simulink model "RobotControl"  (R2016b)
settings: Solver=FixedStepDiscrete  StartTime=0.0  StopTime=inf  FixedStep=0.001  RelTol=1e-3
libraries: arduinolib x9, RobotControlLib x1
settings Model: ExtModeTrigDuration=2  Creator=oelkawok  LastModifiedBy=oelkawok
settings DataIOCC: SaveOutput=off  SaveTime=off
settings OptimizationCC: DefaultParameterBehavior=Inlined  UseFloatMulNetSlope=on  DefaultUnderspecifiedDataType=single  EfficientFloat2IntCast=on  MaxStackSize=64
settings HardwareCC: ProdBitPerInt=16  ProdBitPerPointer=16  ProdBitPerSizeT=16  ProdBitPerPtrDiffT=16  ProdLargestAtomicFloat=None  ProdWordSize=8  ProdHWDeviceType=Atmel->AVR  UseEmbeddedCoderFeatures=off
settings SFSimCC: SimUserSources="\"twi.c\""
settings RTWCC: SystemTargetFile=ert.tlc  GenerateMakefile=off  TemplateMakefile=RTW.MSVCBuild  Description=Create Visual C/C++ Solution File for Embedded Coder  GenerateReport=on  RTWUseSimCustomCode=on  CustomSource="\"twi.c\""  Toolchain=Arduino AVR  BuildConfiguration=Faster Runs  IncludeHyperlinkInReport=on  LaunchReport=on  GenerateTraceInfo=on  GenerateTraceReport=on  GenerateTraceReportSl=on  GenerateTraceReportSf=on  GenerateTraceReportEml=on  GenerateCodeMetricsReport=on
settings CodeAppCC: ForceParamTrailComments=on  IgnoreCustomStorageClasses=off  OperatorAnnotations=on  SimulinkDataObjDesc=on  SFDataObjDesc=on  MATLABFcnDesc=on  InsertBlockDesc=on  MATLABSourceComments=on
settings ERTTargetCC: GenerateSampleERTMain=on  SupportComplex=off  InlinedParameterPlacement=NonHierarchical  ERTCustomFileTemplate=example_file_process.tlc  MemSecPackage=Simulink

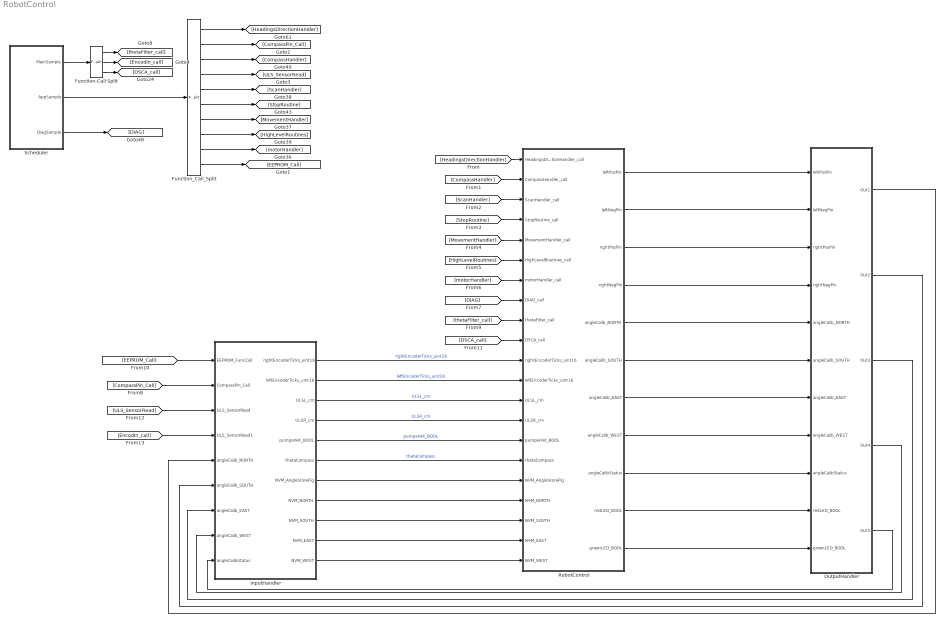
== system RobotControl ==
  Function-Call Split : FunctionCallSplit  IconShape=distinctive  NumOutputPorts=3  OutputPortLayout=default
  Function_Call_Split : FunctionCallSplit  IconShape=distinctive  NumOutputPorts=10  OutputPortLayout=default
  InputHandler : Subsystem
  OutputHandler : Subsystem
  RobotControl : Subsystem
  Scheduler : Subsystem
  wires:
  Scheduler/2(AppSample) -> Function_Call_Split/1
  Function_Call_Split/1 -> [HeadingsDirectionHandler]
  Scheduler/3(DiagSample) -> [DIAG]
  [HeadingsDirectionHandler] -> RobotControl/1(HeadingsDirectionHandler_call)
  [CompassHandler] -> RobotControl/2(CompassHandler_call)
  [ScanHandler] -> RobotControl/3(ScanHandler_call)
  [StopRoutine] -> RobotControl/4(StopRoutine_call)
  [HighLevelRoutines] -> RobotControl/6(HighLevelRoutines_call)
  [MovementHandler] -> RobotControl/5(MovementHandler_call)
  [motorHandler] -> RobotControl/7(motorHandler_call)
  RobotControl/1(leftPosPin) -> OutputHandler/1(leftPosPin)
  RobotControl/2(leftNegPin) -> OutputHandler/2(leftNegPin)
  RobotControl/3(rightPosPin) -> OutputHandler/3(rightPosPin)
  RobotControl/4(rightNegPin) -> OutputHandler/4(rightNegPin)
  RobotControl/5(angleCalib_NORTH) -> OutputHandler/5(angleCalib_NORTH)
  RobotControl/6(angleCalib_SOUTH) -> OutputHandler/6(angleCalib_SOUTH)
  RobotControl/7(angleCalib_EAST) -> OutputHandler/7(angleCalib_EAST)
  RobotControl/8(angleCalib_WEST) -> OutputHandler/8(angleCalib_WEST)
  RobotControl/9(angleCalibStatus) -> OutputHandler/9(angleCalibStatus)
  RobotControl/10(redLED_BOOL) -> OutputHandler/10(redLED_BOOL)
  RobotControl/11(greenLED_BOOL) -> OutputHandler/11(greenLED_BOOL)
  [DIAG] -> RobotControl/8(DIAG_call)
  [EEPROM_Call] -> InputHandler/1(EEPROM_FuncCall)
  OutputHandler/5(Out5) -> InputHandler/9(angleCalibStatus)
  OutputHandler/4(Out4) -> InputHandler/8(angleCalib_WEST)
  OutputHandler/3(Out3) -> InputHandler/7(angleCalib_EAST)
  OutputHandler/2(Out2) -> InputHandler/6(angleCalib_SOUTH)
  OutputHandler/1(Out1) -> InputHandler/5(angleCalib_NORTH)
  [CompassPin_Call] -> InputHandler/2(CompassPin_Call)
  Function_Call_Split/2 -> [CompassPin_Call]
  Function_Call_Split/3 -> [CompassHandler]
  Scheduler/1(MainSample) -> Function-Call Split/1
  Function-Call Split/1 -> [thetaFilter_call]
  [DSCA_call] -> RobotControl/10(DSCA_call)
  [thetaFilter_call] -> RobotControl/9(thetaFilter_call)
  InputHandler/11(NVM_WEST) -> RobotControl/21(NVM_WEST)
  InputHandler/10(NVM_EAST) -> RobotControl/20(NVM_EAST)
  InputHandler/9(NVM_SOUTH) -> RobotControl/19(NVM_SOUTH)
  InputHandler/8(NVM_NORTH) -> RobotControl/18(NVM_NORTH)
  InputHandler/7(NVM_AngleStoreFlg) -> RobotControl/17(NVM_AngleStoreFlg)
  InputHandler/6(thetaCompass) -> RobotControl/16(thetaCompass)  "thetaCompass"
  InputHandler/5(pumperHit_BOOL) -> RobotControl/15(pumperHit_BOOL)  "pumperHit_BOOL"
  InputHandler/4(ULSR_cm) -> RobotControl/14(ULSR_cm)  "ULSR_cm"
  InputHandler/3(ULSL_cm) -> RobotControl/13(ULSL_cm)  "ULSL_cm"
  InputHandler/2(leftEncoderTicks_uint16) -> RobotControl/12(leftEncoderTicks_uint16)  "leftEncoderTicks_uint16"
  InputHandler/1(rightEncoderTicks_uint16) -> RobotControl/11(rightEncoderTicks_uint16)  "rightEncoderTicks_uint16"
  Function_Call_Split/4 -> [ULS_SensorRead]
  Function_Call_Split/5 -> [ScanHandler]
  Function_Call_Split/7 -> [MovementHandler]
  Function_Call_Split/6 -> [StopRoutine]
  Function_Call_Split/8 -> [HighLevelRoutines]
  Function_Call_Split/9 -> [motorHandler]
  Function_Call_Split/10 -> [EEPROM_Call]
  [ULS_SensorRead] -> InputHandler/3(ULS_SensorRead)
  Function-Call Split/3 -> [DSCA_call]
  Function-Call Split/2 -> [EncodIn_call]
  [EncodIn_call] -> InputHandler/4(ULS_SensorRead1)

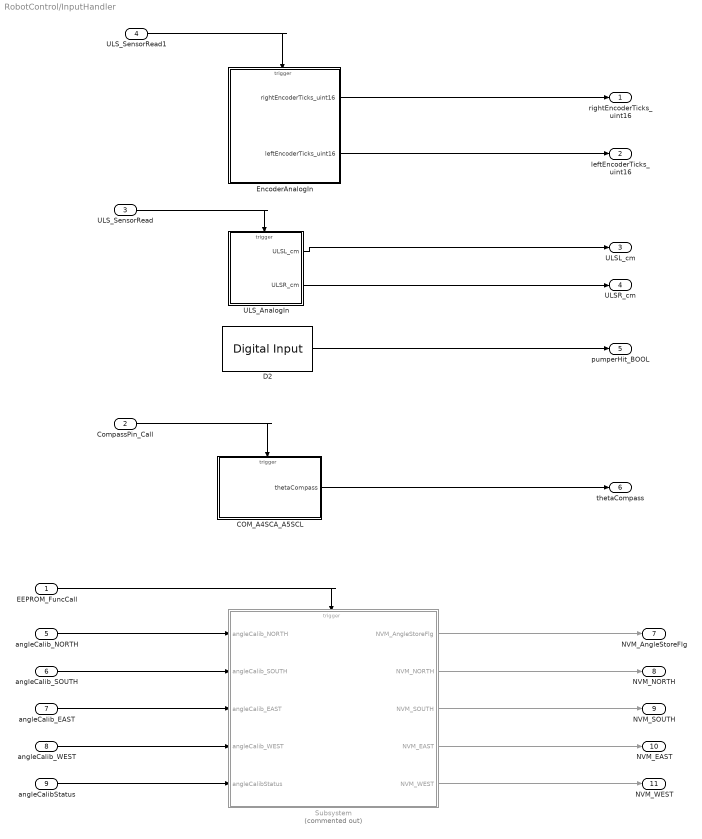
== system RobotControl/InputHandler ==
  EEPROM_FuncCall : Inport
  CompassPin_Call : Inport  Port=2
  ULS_SensorRead : Inport  Port=3
  ULS_SensorRead1 : Inport  Port=4
  angleCalib_NORTH : Inport  Port=5
  angleCalib_SOUTH : Inport  Port=6
  angleCalib_EAST : Inport  Port=7
  angleCalib_WEST : Inport  Port=8
  angleCalibStatus : Inport  Port=9
  COM_A4SCA_A5SCL : Subsystem
      settings: RTWSystemCode=Nonreusable function  RTWFcnNameOpts=Use subsystem name  RTWFileNameOpts=Use subsystem name
  D2 : arduinolib/Digital Input  pinNumber=2  sampleTime=-1  blockPlatform=arduino
  EncoderAnalogIn : Subsystem  RTWFileName=DSCA
      settings: RTWSystemCode=Nonreusable function  RTWFcnNameOpts=Use subsystem name  RTWFileNameOpts=User specified
  Subsystem : Subsystem  Commented=on
  ULS_AnalogIn : Subsystem  RTWFileName=ScanHandler
      settings: ErrorFcn=ScanHandler  RTWSystemCode=Nonreusable function  RTWFcnNameOpts=Use subsystem name  RTWFileNameOpts=User specified
  rightEncoderTicks_uint16 : Outport
  leftEncoderTicks_uint16 : Outport  Port=2
  ULSL_cm : Outport  Port=3
  ULSR_cm : Outport  Port=4
  pumperHit_BOOL : Outport  Port=5
  thetaCompass : Outport  Port=6
  NVM_AngleStoreFlg : Outport  Port=7
  NVM_NORTH : Outport  Port=8
  NVM_SOUTH : Outport  Port=9
  NVM_EAST : Outport  Port=10
  NVM_WEST : Outport  Port=11
  wires:
  D2/1 -> pumperHit_BOOL/1
  EEPROM_FuncCall/1 -> Subsystem/Trigger
  angleCalib_NORTH/1 -> Subsystem/1(angleCalib_NORTH)
  angleCalib_SOUTH/1 -> Subsystem/2(angleCalib_SOUTH)
  angleCalib_EAST/1 -> Subsystem/3(angleCalib_EAST)
  angleCalibStatus/1 -> Subsystem/5(angleCalibStatus)
  angleCalib_WEST/1 -> Subsystem/4(angleCalib_WEST)
  Subsystem/5(NVM_WEST) -> NVM_WEST/1
  Subsystem/4(NVM_EAST) -> NVM_EAST/1
  Subsystem/3(NVM_SOUTH) -> NVM_SOUTH/1
  Subsystem/1(NVM_AngleStoreFlg) -> NVM_AngleStoreFlg/1
  Subsystem/2(NVM_NORTH) -> NVM_NORTH/1
  COM_A4SCA_A5SCL/1(thetaCompass) -> thetaCompass/1
  CompassPin_Call/1 -> COM_A4SCA_A5SCL/Trigger
  ULS_AnalogIn/1(ULSL_cm) -> ULSL_cm/1
  ULS_AnalogIn/2(ULSR_cm) -> ULSR_cm/1
  ULS_SensorRead/1 -> ULS_AnalogIn/Trigger
  EncoderAnalogIn/1(rightEncoderTicks_uint16) -> rightEncoderTicks_uint16/1
  EncoderAnalogIn/2(leftEncoderTicks_uint16) -> leftEncoderTicks_uint16/1
  ULS_SensorRead1/1 -> EncoderAnalogIn/Trigger

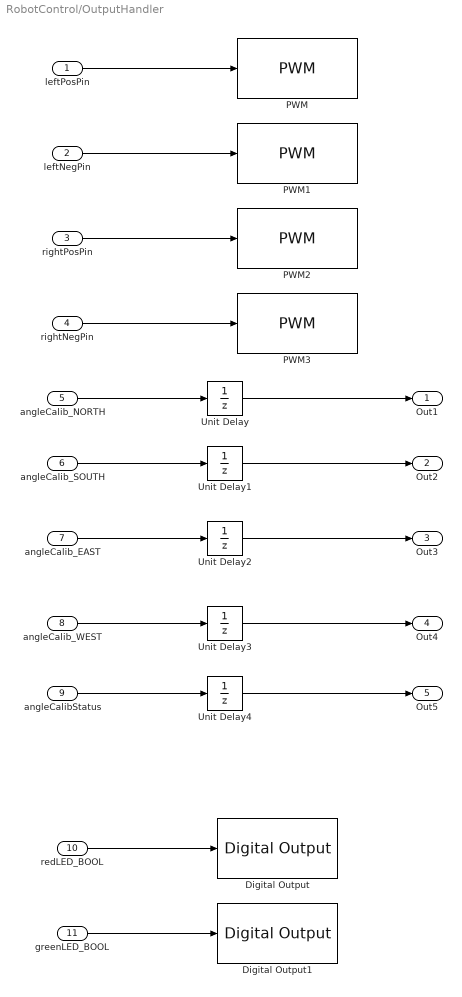
== system RobotControl/OutputHandler ==
  leftPosPin : Inport
  leftNegPin : Inport  Port=2
  rightPosPin : Inport  Port=3
  rightNegPin : Inport  Port=4
  angleCalib_NORTH : Inport  Port=5
  angleCalib_SOUTH : Inport  Port=6
  angleCalib_EAST : Inport  Port=7
  angleCalib_WEST : Inport  Port=8
  angleCalibStatus : Inport  Port=9
  redLED_BOOL : Inport  Port=10
  greenLED_BOOL : Inport  Port=11
  Digital Output : arduinolib/Digital Output  pinNumber=3  blockPlatform=arduino
  Digital Output1 : arduinolib/Digital Output  pinNumber=11  blockPlatform=arduino
  PWM : arduinolib/PWM  pinNumber=5  blockPlatform=arduino
  PWM1 : arduinolib/PWM  pinNumber=6  blockPlatform=arduino
  PWM2 : arduinolib/PWM  pinNumber=9  blockPlatform=arduino
  PWM3 : arduinolib/PWM  pinNumber=10  blockPlatform=arduino
  Unit Delay{,1..4} (5 alike) : UnitDelay  SampleTime=-1
  Out1 : Outport
  Out2 : Outport  Port=2
  Out3 : Outport  Port=3
  Out4 : Outport  Port=4
  Out5 : Outport  Port=5
  wires:
  angleCalib_NORTH/1 -> Unit Delay/1
  angleCalib_SOUTH/1 -> Unit Delay1/1
  angleCalib_WEST/1 -> Unit Delay3/1
  angleCalib_EAST/1 -> Unit Delay2/1
  angleCalibStatus/1 -> Unit Delay4/1
  Unit Delay/1 -> Out1/1
  Unit Delay1/1 -> Out2/1
  Unit Delay3/1 -> Out4/1
  Unit Delay2/1 -> Out3/1
  Unit Delay4/1 -> Out5/1
  leftPosPin/1 -> PWM/1
  leftNegPin/1 -> PWM1/1
  rightPosPin/1 -> PWM2/1
  rightNegPin/1 -> PWM3/1
  redLED_BOOL/1 -> Digital Output/1
  greenLED_BOOL/1 -> Digital Output1/1

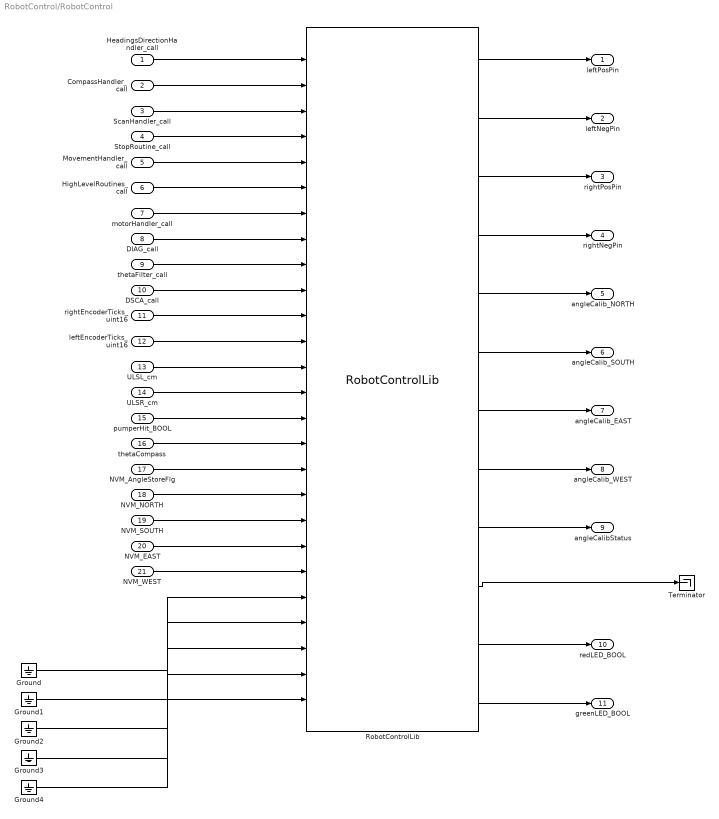
== system RobotControl/RobotControl ==
  HeadingsDirectionHandler_call : Inport  PortDimensions=1
  CompassHandler_call : Inport  Port=2  PortDimensions=1
  ScanHandler_call : Inport  Port=3  PortDimensions=1
  StopRoutine_call : Inport  Port=4  PortDimensions=1
  MovementHandler_call : Inport  Port=5  PortDimensions=1
  HighLevelRoutines_call : Inport  Port=6  PortDimensions=1
  motorHandler_call : Inport  Port=7  PortDimensions=1
  DIAG_call : Inport  Port=8  PortDimensions=1
  thetaFilter_call : Inport  Port=9  PortDimensions=1
  DSCA_call : Inport  Port=10  PortDimensions=1
  rightEncoderTicks_uint16 : Inport  Port=11  PortDimensions=1
  leftEncoderTicks_uint16 : Inport  Port=12  PortDimensions=1
  ULSL_cm : Inport  Port=13  PortDimensions=1
  ULSR_cm : Inport  Port=14  PortDimensions=1
  pumperHit_BOOL : Inport  Port=15  OutDataTypeStr=boolean  PortDimensions=1
  thetaCompass : Inport  Port=16  OutDataTypeStr=int16  PortDimensions=1
  NVM_AngleStoreFlg : Inport  Port=17  PortDimensions=1
  NVM_NORTH : Inport  Port=18  PortDimensions=1
  NVM_SOUTH : Inport  Port=19  PortDimensions=1
  NVM_EAST : Inport  Port=20  PortDimensions=1
  NVM_WEST : Inport  Port=21  PortDimensions=1
  Ground{,1..4} (5 alike) : Ground
  RobotControlLib : RobotControlLib/RobotControlLib
  Terminator : Terminator
  leftPosPin : Outport  OutDataTypeStr=uint8  PortDimensions=1
      settings: AttributesFormatString=|
      | Mode: %<OutputWhenDisabled>
      | Init: %<InitialOutput>
  leftNegPin : Outport  Port=2  OutDataTypeStr=uint8  PortDimensions=1
      settings: AttributesFormatString=|
      | Mode: %<OutputWhenDisabled>
      | Init: %<InitialOutput>
  rightPosPin : Outport  Port=3  OutDataTypeStr=uint8  PortDimensions=1
      settings: AttributesFormatString=|
      | Mode: %<OutputWhenDisabled>
      | Init: %<InitialOutput>
  rightNegPin : Outport  Port=4  OutDataTypeStr=uint8  PortDimensions=1
      settings: AttributesFormatString=|
      | Mode: %<OutputWhenDisabled>
      | Init: %<InitialOutput>
  angleCalib_NORTH : Outport  Port=5  InitialOutput=0
      settings: AttributesFormatString=|
      | Mode: %<OutputWhenDisabled>
      | Init: %<InitialOutput>
  angleCalib_SOUTH : Outport  Port=6  InitialOutput=0
      settings: AttributesFormatString=|
      | Mode: %<OutputWhenDisabled>
      | Init: %<InitialOutput>
  angleCalib_EAST : Outport  Port=7  InitialOutput=0
      settings: AttributesFormatString=|
      | Mode: %<OutputWhenDisabled>
      | Init: %<InitialOutput>
  angleCalib_WEST : Outport  Port=8  InitialOutput=0
      settings: AttributesFormatString=|
      | Mode: %<OutputWhenDisabled>
      | Init: %<InitialOutput>
  angleCalibStatus : Outport  Port=9
      settings: AttributesFormatString=|
      | Mode: %<OutputWhenDisabled>
      | Init: %<InitialOutput>
  redLED_BOOL : Outport  Port=10
      settings: AttributesFormatString=|
      | Mode: %<OutputWhenDisabled>
      | Init: %<InitialOutput>
  greenLED_BOOL : Outport  Port=11
      settings: AttributesFormatString=|
      | Mode: %<OutputWhenDisabled>
      | Init: %<InitialOutput>
  wires:
  RobotControlLib/5 -> angleCalib_NORTH/1
  RobotControlLib/6 -> angleCalib_SOUTH/1
  RobotControlLib/7 -> angleCalib_EAST/1
  RobotControlLib/8 -> angleCalib_WEST/1
  RobotControlLib/4 -> rightNegPin/1
  RobotControlLib/3 -> rightPosPin/1
  RobotControlLib/2 -> leftNegPin/1
  RobotControlLib/1 -> leftPosPin/1
  RobotControlLib/11 -> redLED_BOOL/1
  RobotControlLib/12 -> greenLED_BOOL/1
  RobotControlLib/9 -> angleCalibStatus/1
  RobotControlLib/10 -> Terminator/1
  ScanHandler_call/1 -> RobotControlLib/3
  CompassHandler_call/1 -> RobotControlLib/2
  StopRoutine_call/1 -> RobotControlLib/4
  HeadingsDirectionHandler_call/1 -> RobotControlLib/1
  MovementHandler_call/1 -> RobotControlLib/5
  HighLevelRoutines_call/1 -> RobotControlLib/6
  motorHandler_call/1 -> RobotControlLib/7
  DIAG_call/1 -> RobotControlLib/8
  thetaFilter_call/1 -> RobotControlLib/9
  DSCA_call/1 -> RobotControlLib/10
  rightEncoderTicks_uint16/1 -> RobotControlLib/11
  leftEncoderTicks_uint16/1 -> RobotControlLib/12
  ULSL_cm/1 -> RobotControlLib/13
  ULSR_cm/1 -> RobotControlLib/14
  pumperHit_BOOL/1 -> RobotControlLib/15
  thetaCompass/1 -> RobotControlLib/16
  NVM_AngleStoreFlg/1 -> RobotControlLib/17
  NVM_NORTH/1 -> RobotControlLib/18
  NVM_SOUTH/1 -> RobotControlLib/19
  NVM_EAST/1 -> RobotControlLib/20
  NVM_WEST/1 -> RobotControlLib/21
  Ground/1 -> RobotControlLib/22
  Ground1/1 -> RobotControlLib/23
  Ground2/1 -> RobotControlLib/24
  Ground3/1 -> RobotControlLib/25
  Ground4/1 -> RobotControlLib/26

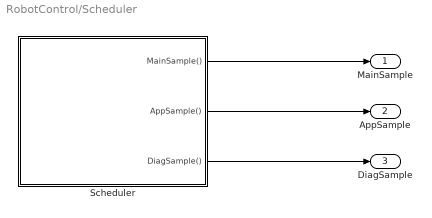
== system RobotControl/Scheduler ==
  Scheduler : Stateflow chart  TreatAsAtomicUnit=on
  MainSample : Outport
  AppSample : Outport  Port=2
  DiagSample : Outport  Port=3
  wires:
  Scheduler/3(DiagSample()) -> DiagSample/1
  Scheduler/2(AppSample()) -> AppSample/1
  Scheduler/1(MainSample()) -> MainSample/1

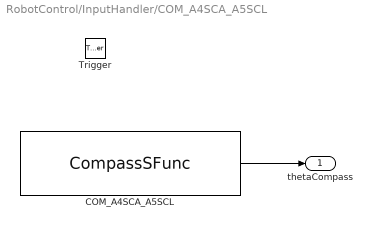
== system RobotControl/InputHandler/COM_A4SCA_A5SCL ==
  Trigger : TriggerPort  TriggerType=function-call  VariantControl=Variant  PortDimensions=1
  COM_A4SCA_A5SCL : S-Function  InitFcn=try, set_param(gcb,'FunctionName','CompassSFunc'), end  FunctionName=CompassSFunc  SFunctionModules=CompassSFunc_wrapper  SFunctionDeploymentMode=off  EnableBusSupport=off  mask(S-Function Builder){}
      mask help: Simulink:masks:SFunctionBuilder_MD
      mask init:
      | val = [[.9  0.75 0.75 1 1 .9 .9 1]',[1 1 0.75 0.75 .9 .9 1 .9]'];try , sys = get_param(gcb,'SfunBuilderFcnName');if isempty(sys), sys = get_param(gcb,'FunctionName'); end,catch, sys = get_param(gcb,'FunctionName'); end
      settings: CopyFcn=set_param(gcbh,'LinkStatus','none')  PreSaveFcn=try, set_param(gcb,'FunctionName','CompassSFunc'), end  OpenFcn=sfunctionwizard(gcbh)
      mask Display: plot(val(:,1),val(:,2)),disp(sys), port_label('output',1,'Temp_angle')
  thetaCompass : Outport
  wires:
  COM_A4SCA_A5SCL/1 -> thetaCompass/1

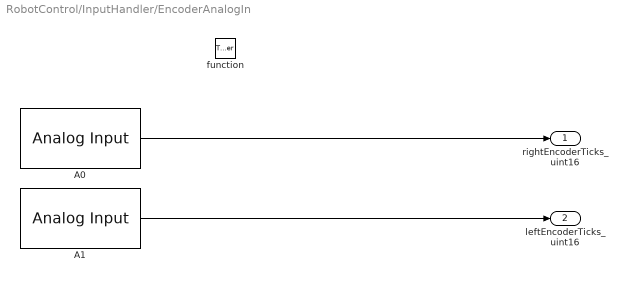
== system RobotControl/InputHandler/EncoderAnalogIn ==
  function : TriggerPort  TriggerType=function-call  VariantControl=Variant
  A0 : arduinolib/Analog Input  pinNumber=0  sampleTime=-1  blockPlatform=arduino
  A1 : arduinolib/Analog Input  pinNumber=1  sampleTime=-1  blockPlatform=arduino
  rightEncoderTicks_uint16 : Outport
  leftEncoderTicks_uint16 : Outport  Port=2
  wires:
  A1/1 -> leftEncoderTicks_uint16/1
  A0/1 -> rightEncoderTicks_uint16/1

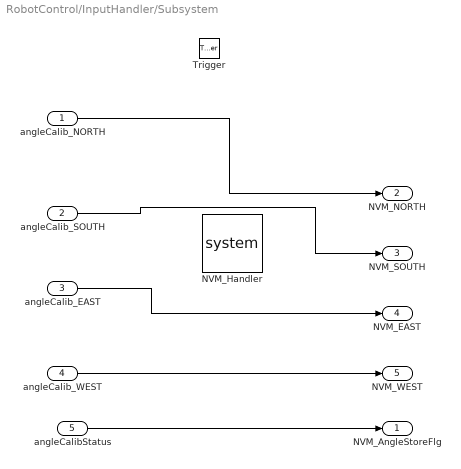
== system RobotControl/InputHandler/Subsystem ==
  angleCalib_NORTH : Inport
  angleCalib_SOUTH : Inport  Port=2
  angleCalib_EAST : Inport  Port=3
  angleCalib_WEST : Inport  Port=4
  angleCalibStatus : Inport  Port=5
  Trigger : TriggerPort  TriggerType=function-call  VariantControl=Variant  PortDimensions=1
  NVM_Handler : S-Function  SFunctionDeploymentMode=off  EnableBusSupport=off  mask(S-Function Builder){}
      mask help: Simulink:masks:SFunctionBuilder_MD
      mask init:
      | val = [[.9  0.75 0.75 1 1 .9 .9 1]',[1 1 0.75 0.75 .9 .9 1 .9]'];
      | sys = get_param(gcbh,'FunctionName');
      settings: CopyFcn=set_param(gcbh,'LinkStatus','none')  OpenFcn=sfunctionwizard(gcbh)
      mask Display:
      | plot(val(:,1),val(:,2))
      | disp(sys)
  NVM_AngleStoreFlg : Outport
  NVM_NORTH : Outport  Port=2
  NVM_SOUTH : Outport  Port=3
  NVM_EAST : Outport  Port=4
  NVM_WEST : Outport  Port=5
  wires:
  angleCalib_NORTH/1 -> NVM_NORTH/1
  angleCalib_SOUTH/1 -> NVM_SOUTH/1
  angleCalib_EAST/1 -> NVM_EAST/1
  angleCalib_WEST/1 -> NVM_WEST/1
  angleCalibStatus/1 -> NVM_AngleStoreFlg/1

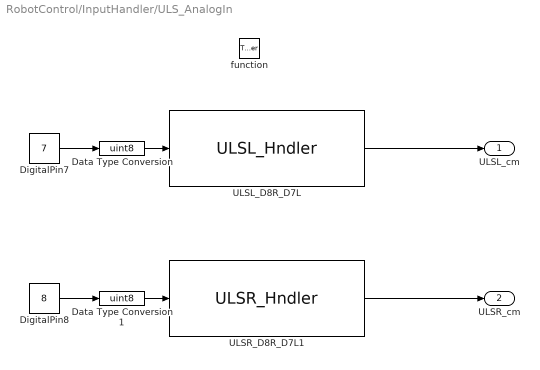
== system RobotControl/InputHandler/ULS_AnalogIn ==
  function : TriggerPort  TriggerType=function-call  VariantControl=Variant
  Data Type Conversion : DataTypeConversion  OutDataTypeStr=uint8
  Data Type Conversion1 : DataTypeConversion  OutDataTypeStr=uint8
  DigitalPin7 : Constant  Value=7
  DigitalPin8 : Constant  Value=8
  ULSL_D8R_D7L : S-Function  InitFcn=try, set_param(gcb,'FunctionName','ULSL_Hndler'), end  FunctionName=ULSL_Hndler  SFunctionModules=ULSL_Hndler_wrapper  SFunctionDeploymentMode=off  EnableBusSupport=off  mask(S-Function Builder){}
      mask help: Simulink:masks:SFunctionBuilder_MD
      mask init: same as RobotControl/InputHandler/COM_A4SCA_A5SCL/COM_A4SCA_A5SCL
      settings: CopyFcn=set_param(gcbh,'LinkStatus','none')  PreSaveFcn=try, set_param(gcb,'FunctionName','ULSL_Hndler'), end  OpenFcn=sfunctionwizard(gcbh)
      mask Display: plot(val(:,1),val(:,2)),disp(sys), port_label('input',1,'ULSL_Pin'), port_label('output',1,'ULSL_cm')
  ULSR_D8R_D7L1 : S-Function  InitFcn=try, set_param(gcb,'FunctionName','ULSR_Hndler'), end  FunctionName=ULSR_Hndler  SFunctionModules=ULSR_Hndler_wrapper  SFunctionDeploymentMode=off  EnableBusSupport=off  mask(S-Function Builder){}
      mask help: Simulink:masks:SFunctionBuilder_MD
      mask init: same as RobotControl/InputHandler/COM_A4SCA_A5SCL/COM_A4SCA_A5SCL
      settings: CopyFcn=set_param(gcbh,'LinkStatus','none')  PreSaveFcn=try, set_param(gcb,'FunctionName','ULSR_Hndler'), end  OpenFcn=sfunctionwizard(gcbh)
      mask Display: plot(val(:,1),val(:,2)),disp(sys), port_label('input',1,'ULSR_Pin'), port_label('output',1,'ULSR_cm')
  ULSL_cm : Outport
  ULSR_cm : Outport  Port=2
  wires:
  ULSL_D8R_D7L/1 -> ULSL_cm/1
  Data Type Conversion1/1 -> ULSR_D8R_D7L1/1
  DigitalPin7/1 -> Data Type Conversion/1
  DigitalPin8/1 -> Data Type Conversion1/1
  Data Type Conversion/1 -> ULSL_D8R_D7L/1
  ULSR_D8R_D7L1/1 -> ULSR_cm/1

== stateflow chart RobotControl/Scheduler/Scheduler ==
  settings: description=scheduler for the SWCs
  state Scheduler
    //every 1ms
    du:
    send(MainSample);
    //every 5ms
    on every(CAL_APP_Ticks_Sec, tick):
    send(AppSample);
    //every 50ms
    on every(CAL_DIAG_Ticks_Sec, tick):
    send(DiagSample);
  data: CAL_APP_Ticks_Sec constant uint8 =CAL_APP_Ticks_Sec; CAL_DIAG_Ticks_Sec constant uint8 =CAL_DIAG_Ticks_Sec
  events: MainSample output FUNCTION_CALL_EVENT; AppSample output FUNCTION_CALL_EVENT; DiagSample output FUNCTION_CALL_EVENT
